simulink model "Elemnts"  (R2019a)
settings: Solver=VariableStepAuto  StartTime=0.0  StopTime=""  RelTol=1e-3
libraries: powerlib_meascontrol x6, powerlib x6
settings Model: Creator=Night_Bird  LastModifiedBy=Night_Bird

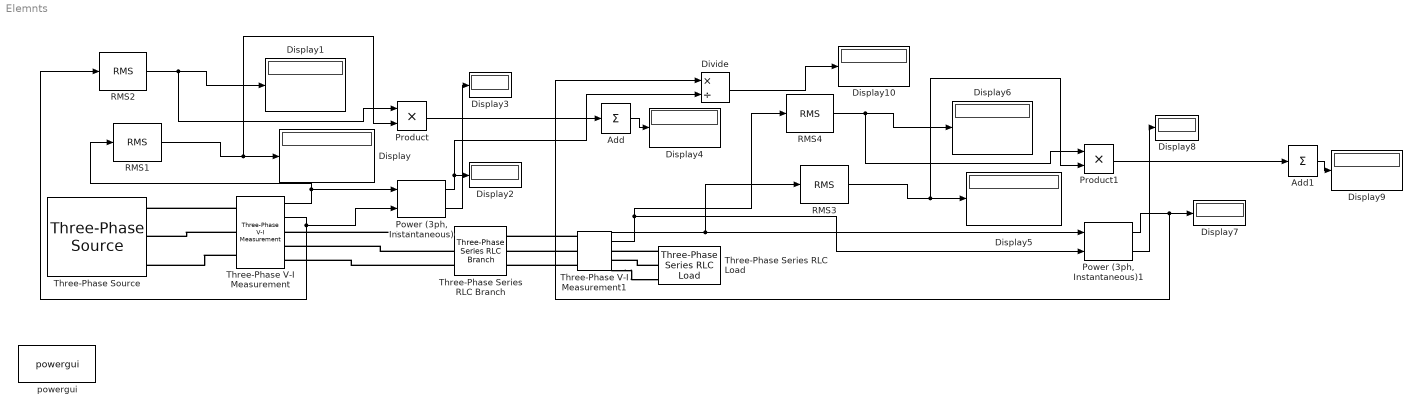
== system Elemnts ==
  Add : Sum  Inputs=+
  Add1 : Sum  Inputs=+
  Display{,1..10} (11 alike) : Display
  Divide : Product  Inputs=*/
  "Power (3ph, Instantaneous)" : powerlib_meascontrol/Measurements/Power (3ph, Instantaneous)
      settings: SourceProductName=Simscape Electrical
  "Power (3ph, Instantaneous)1" : powerlib_meascontrol/Measurements/Power (3ph, Instantaneous)
      settings: SourceProductName=Simscape Electrical
  Product : Product
  Product1 : Product
  RMS{1..4} (4 alike) : powerlib_meascontrol/Measurements/RMS  TrueRMS=on  Freq=60  RMSInit=0  Ts=0
      settings: SourceProductName=Simscape Electrical
  Three-Phase Series RLC Branch : powerlib/Elements/Three-Phase Series RLC Branch  LConnTagsString=A|B|C  RConnTagsString=A|B|C  BranchType=RL  Resistance=10  Inductance=1e-3  Capacitance=1e-6  Measurements=None
      settings: SourceProductName=Simscape Electrical
  Three-Phase Series RLC Load : powerlib/Elements/Three-Phase Series RLC Load  LConnTagsString=A|B|C  Configuration=Y (grounded)  NominalVoltage=250e3  Vabc=[1e3 1e3 1e3]  Vabcp=[1e3 1e3 1e3]  NominalFrequency=60  UnbalancedPower=off  ActivePower=10e3  InductivePower=220e6  CapacitivePower=0  Pabc=[10e3 9e3 11e3]  QLabc=[100 90 110]  QCabc=[100 90 110]  Pabcp=[10e3 9e3 11e3]  QLabcp=[100 90 110]  QCabcp=[100 90 110]  Measurements=None  LoadType=constant Z
      settings: SourceProductName=Simscape Electrical
  Three-Phase V-I Measurement : powerlib/Measurements/Three-Phase V-I Measurement  VoltageMeasurement=phase-to-ground  SetLabelV=off  LabelV=Vabc  Vpu=off  VpuLL=off  CurrentMeasurement=yes  SetLabelI=off  LabelI=Iabc  Ipu=off  Pbase=100e6  Vbase=500e3  OutputType=Complex  PhasorSimulation=off  PSBequivalent=0
      settings: SourceProductName=Simscape Electrical
  Three-Phase V-I Measurement1 : powerlib/Measurements/Three-Phase V-I Measurement  VoltageMeasurement=phase-to-ground  SetLabelV=off  LabelV=Vabc  Vpu=off  VpuLL=off  CurrentMeasurement=yes  SetLabelI=off  LabelI=Iabc  Ipu=off  Pbase=100e6  Vbase=500e3  OutputType=Complex  PhasorSimulation=off  PSBequivalent=0
      settings: SourceProductName=Simscape Electrical
  Three-Phase Source : powerlib/Electrical Sources/Three-Phase Source  InternalConnection=Yg  VoltagePhases=off  Voltage=250e3  PhaseAngle=0  Voltage_phases=[25e3 25e3 25e3]/sqrt(3)  PhaseAngles_phases=[0 -120 +120]  Frequency=60  NonIdealSource=off  SpecifyImpedance=off  Resistance=0.8929  Inductance=16.58e-3  ShortCircuitLevel=100e6  BaseVoltage=25e3  XRratio=7  BusType=swing  Pref=10e3  Qref=0  Prefabc=[10e3, 10e3, 10e3]  Qrefabc=[0, 0, 0]  Qmin=-inf  Qmax=inf
      settings: SourceProductName=Simscape Electrical
  powergui : powerlib/powergui  Priority=1  SimulationMode=Continuous  SampleTime=50e-6  frequency=60  Iterations=50  frequencyindice=60  Pbase=100e6  ErrMax=1e-4  UnitsV=kV  UnitsW=MW  buscounter=0  FunctionMessages=off  echomessages=off  EnableUseOfTLC=off  CurrentSourceSwitches=off  DisableSnubberDevices=off  DisableRonSwitches=off  DisableVfSwitches=off  DisplayEquations=off  AutomaticDiscreteSolvers=off  SolverType=Tustin/Backward Euler (TBE)  Interpol=off  ExternalGateDelay=off  methode=off  Ts=100  x0status=blocks  SPID=on  SwTol=0  HookPort=off  NonlinearTolerance=0  nMaxIteration=15  ContinueOnMaxIteration=off  RestoreLinks=warning  ResistiveCurrentMeasurement=off  Frange=[0:2:500]  Ylog=off  Xlog=on  ShowGrid=off  save=off  variable=ZData  structure=0  ZoomFFT=off  StartTime=0.0  cycles=1  DisplayStyle=1  fundamental=60  FreqAxis=off  MaxFrequency=1000  frequencyindicesteady=1  RmsSteady=1  display=off
      settings: SourceProductName=Simscape Electrical
  wires:
  Three-Phase V-I Measurement/1 -> "Power (3ph, Instantaneous)"/1, RMS1/1
  RMS1/1 -> Product/2, Display/1
  RMS2/1 -> Product/1, Display1/1
  Three-Phase V-I Measurement/2 -> "Power (3ph, Instantaneous)"/2, RMS2/1
  "Power (3ph, Instantaneous)"/1 -> Divide/2, Display2/1
  "Power (3ph, Instantaneous)"/2 -> Display3/1
  Product/1 -> Add/1
  Add/1 -> Display4/1
  RMS3/1 -> Product1/2, Display5/1
  Product1/1 -> Add1/1
  "Power (3ph, Instantaneous)1"/1 -> Divide/1, Display7/1
  "Power (3ph, Instantaneous)1"/2 -> Display8/1
  RMS4/1 -> Product1/1, Display6/1
  Add1/1 -> Display9/1
  Three-Phase V-I Measurement1/1 -> RMS3/1, "Power (3ph, Instantaneous)1"/1
  Three-Phase V-I Measurement1/2 -> "Power (3ph, Instantaneous)1"/2, RMS4/1
  Divide/1 -> Display10/1
  connections:
  Three-Phase V-I Measurement/LConn3 -- Three-Phase Source/RConn3
  Three-Phase V-I Measurement/LConn2 -- Three-Phase Source/RConn2
  Three-Phase V-I Measurement/LConn1 -- Three-Phase Source/RConn1
  Three-Phase Series RLC Branch/LConn1 -- Three-Phase V-I Measurement/RConn1
  Three-Phase Series RLC Branch/LConn2 -- Three-Phase V-I Measurement/RConn2
  Three-Phase Series RLC Branch/LConn3 -- Three-Phase V-I Measurement/RConn3
  Three-Phase V-I Measurement1/LConn1 -- Three-Phase Series RLC Branch/RConn1
  Three-Phase V-I Measurement1/LConn2 -- Three-Phase Series RLC Branch/RConn2
  Three-Phase V-I Measurement1/LConn3 -- Three-Phase Series RLC Branch/RConn3
  Three-Phase Series RLC Load/LConn1 -- Three-Phase V-I Measurement1/RConn1
  Three-Phase Series RLC Load/LConn2 -- Three-Phase V-I Measurement1/RConn2
  Three-Phase V-I Measurement1/RConn3 -- Three-Phase Series RLC Load/LConn3
